simulink model "ForwardSpeedModel"  (Simulink 8.5)
settings: Solver=ode45  StartTime=0.0  StopTime=tstop  RelTol=1e-3
values from neighbouring files (symbols this model uses):
  d_1 = d(1)    [run_task_1_8.m]
  d_2 = d(2)    [run_task_1_8.m]
  m_u = 6000    [run_task_1_8.m]
  n_c = u(2)    [msfartoystyring.m]    (also in run_task_1_8.m = 7.3)
  tsamp = 10    [run_task_1_8.m]
  v0 = [u_r_0 0]'    [run_task_1_8.m]
settings Model: Creator=ONL  LastModifiedBy=ONL
settings DataIOCC: SignalLoggingSaveFormat=Dataset
settings OptimizationCC: ExpressionDepthLimit=128
settings DebuggingCC: UnderspecifiedInitializationDetection=Simplified  MergeDetectMultiDrivingBlocksExec=error  FcnCallInpInsideContextMsg=EnableAllAsError  StateNameClashWarn=none
settings GRTTargetCC: CombineOutputUpdateFcns=on  GRTInterface=off

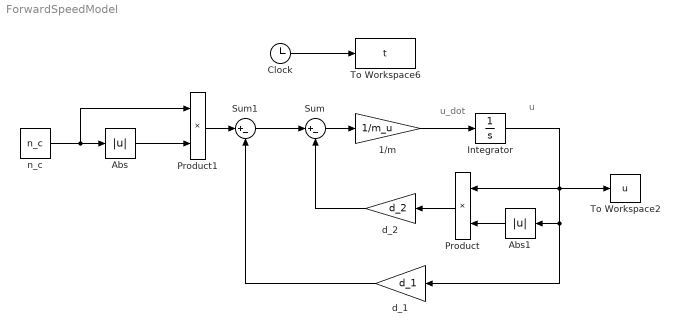
== system ForwardSpeedModel ==
  note: u
  note: u_dot
  1/m : Gain  Gain=1/m_u
  Abs : Abs
  Abs1 : Abs
  Clock : Clock
  Integrator : Integrator  InitialCondition=v0(1)
  Product : Product
  Product1 : Product
  Sum : Sum  Inputs=|+-
  Sum1 : Sum  Inputs=|+-
  To Workspace2 : ToWorkspace  VariableName=u  SampleTime=tsamp
  To Workspace6 : ToWorkspace  VariableName=t  SampleTime=tsamp
  d_1 : Gain  Gain=d_1
  d_2 : Gain  Gain=d_2
  n_c : Constant  Value=n_c
  wires:
  Clock/1 -> To Workspace6/1
  Integrator/1 -> To Workspace2/1, Product/1, d_1/1, Abs1/1
  n_c/1 -> Product1/1, Abs/1
  Abs/1 -> Product1/2
  1/m/1 -> Integrator/1
  Sum/1 -> 1/m/1
  Sum1/1 -> Sum/1
  Product/1 -> d_2/1
  Abs1/1 -> Product/2
  Product1/1 -> Sum1/1
  d_2/1 -> Sum/2
  d_1/1 -> Sum1/2
